simulink model "gps1"  (Simulink 7.5)
settings: Solver=ode45  StartTime=0.0  StopTime=10.0  RelTol=1e-3
undefined symbols (not defined in the file or in its folder): magnitude, serial
libraries: dspsrcs4 x32, dspxfrm3 x4, dsparch4 x2, powerlib_extras x2, dspsigops x2, instrumentlib x2, tiiqmathlib x1
settings Model: Creator=sisa  LastModifiedBy=SISA

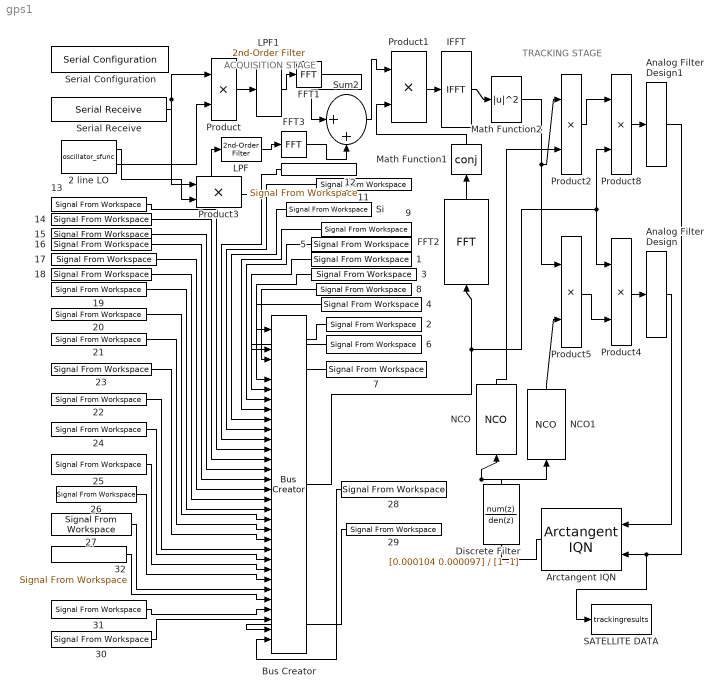
== system gps1 ==
  note: ACQUISITION STAGE
  note: TRACKING STAGE
  1 : dspsrcs4/Signal From Workspace  SystemSampleTime=-1  X=PN07  Ts=1  nsamps=1  OutputAfterFinalValue=Setting to zero  ignoreOrWarnInputAndFrameLengths=off
  11 : dspsrcs4/Signal From Workspace  SystemSampleTime=-1  X=PN11  Ts=1  nsamps=1  OutputAfterFinalValue=Setting to zero  ignoreOrWarnInputAndFrameLengths=off
  12 : dspsrcs4/Signal From Workspace  SystemSampleTime=-1  X=PN12  Ts=1  nsamps=1  OutputAfterFinalValue=Setting to zero  ignoreOrWarnInputAndFrameLengths=off
  13 : dspsrcs4/Signal From Workspace  SystemSampleTime=-1  X=PN13  Ts=1  nsamps=1  OutputAfterFinalValue=Setting to zero  ignoreOrWarnInputAndFrameLengths=off
  14 : dspsrcs4/Signal From Workspace  SystemSampleTime=-1  X=PN14  Ts=1  nsamps=1  OutputAfterFinalValue=Setting to zero  ignoreOrWarnInputAndFrameLengths=off
  15 : dspsrcs4/Signal From Workspace  SystemSampleTime=-1  X=PN15  Ts=1  nsamps=1  OutputAfterFinalValue=Setting to zero  ignoreOrWarnInputAndFrameLengths=off
  16 : dspsrcs4/Signal From Workspace  SystemSampleTime=-1  X=PN16  Ts=1  nsamps=1  OutputAfterFinalValue=Setting to zero  ignoreOrWarnInputAndFrameLengths=off
  17 : dspsrcs4/Signal From Workspace  SystemSampleTime=-1  X=PN17  Ts=1  nsamps=1  OutputAfterFinalValue=Setting to zero  ignoreOrWarnInputAndFrameLengths=off
  18 : dspsrcs4/Signal From Workspace  SystemSampleTime=-1  X=PN18  Ts=1  nsamps=1  OutputAfterFinalValue=Setting to zero  ignoreOrWarnInputAndFrameLengths=off
  19 : dspsrcs4/Signal From Workspace  SystemSampleTime=-1  X=PN19  Ts=1  nsamps=1  OutputAfterFinalValue=Setting to zero  ignoreOrWarnInputAndFrameLengths=off
  2 : dspsrcs4/Signal From Workspace  SystemSampleTime=-1  X=PN03  Ts=1  nsamps=1  OutputAfterFinalValue=Setting to zero  ignoreOrWarnInputAndFrameLengths=off
  2 line LO : M-S-Function  FunctionName=oscillator_sfunc  Parameters=1/38192000
  20 : dspsrcs4/Signal From Workspace  SystemSampleTime=-1  X=PN20  Ts=1  nsamps=1  OutputAfterFinalValue=Setting to zero  ignoreOrWarnInputAndFrameLengths=off
  21 : dspsrcs4/Signal From Workspace  SystemSampleTime=-1  X=PN21  Ts=1  nsamps=1  OutputAfterFinalValue=Setting to zero  ignoreOrWarnInputAndFrameLengths=off
  22 : dspsrcs4/Signal From Workspace  SystemSampleTime=-1  X=PN23  Ts=1  nsamps=1  OutputAfterFinalValue=Setting to zero  ignoreOrWarnInputAndFrameLengths=off
  23 : dspsrcs4/Signal From Workspace  SystemSampleTime=-1  X=PN22  Ts=1  nsamps=1  OutputAfterFinalValue=Setting to zero  ignoreOrWarnInputAndFrameLengths=off
  24 : dspsrcs4/Signal From Workspace  SystemSampleTime=-1  X=PN24  Ts=1  nsamps=1  OutputAfterFinalValue=Setting to zero  ignoreOrWarnInputAndFrameLengths=off
  25 : dspsrcs4/Signal From Workspace  SystemSampleTime=-1  X=PN25  Ts=1  nsamps=1  OutputAfterFinalValue=Setting to zero  ignoreOrWarnInputAndFrameLengths=off
  26 : dspsrcs4/Signal From Workspace  SystemSampleTime=-1  X=PN26  Ts=1  nsamps=1  OutputAfterFinalValue=Setting to zero  ignoreOrWarnInputAndFrameLengths=off
  27 : dspsrcs4/Signal From Workspace  SystemSampleTime=-1  X=PN27  Ts=1  nsamps=1  OutputAfterFinalValue=Setting to zero  ignoreOrWarnInputAndFrameLengths=off
  28 : dspsrcs4/Signal From Workspace  SystemSampleTime=-1  X=PN28  Ts=1  nsamps=1  OutputAfterFinalValue=Setting to zero  ignoreOrWarnInputAndFrameLengths=off
  29 : dspsrcs4/Signal From Workspace  SystemSampleTime=-1  X=PN29  Ts=1  nsamps=1  OutputAfterFinalValue=Setting to zero  ignoreOrWarnInputAndFrameLengths=off
  3 : dspsrcs4/Signal From Workspace  SystemSampleTime=-1  X=PN06  Ts=1  nsamps=1  OutputAfterFinalValue=Setting to zero  ignoreOrWarnInputAndFrameLengths=off
  30 : dspsrcs4/Signal From Workspace  SystemSampleTime=-1  X=PN30  Ts=1  nsamps=1  OutputAfterFinalValue=Setting to zero  ignoreOrWarnInputAndFrameLengths=off
  31 : dspsrcs4/Signal From Workspace  SystemSampleTime=-1  X=PN31  Ts=1  nsamps=1  OutputAfterFinalValue=Setting to zero  ignoreOrWarnInputAndFrameLengths=off
  32 : dspsrcs4/Signal From Workspace  SystemSampleTime=-1  X=PN32  Ts=1  nsamps=1  OutputAfterFinalValue=Setting to zero  ignoreOrWarnInputAndFrameLengths=off
  4 : dspsrcs4/Signal From Workspace  SystemSampleTime=-1  X=PN04  Ts=1  nsamps=1  OutputAfterFinalValue=Setting to zero  ignoreOrWarnInputAndFrameLengths=off
  5 : dspsrcs4/Signal From Workspace  SystemSampleTime=-1  X=PN08  Ts=1  nsamps=1  OutputAfterFinalValue=Setting to zero  ignoreOrWarnInputAndFrameLengths=off
  6 : dspsrcs4/Signal From Workspace  SystemSampleTime=-1  X=PN02  Ts=1  nsamps=1  OutputAfterFinalValue=Setting to zero  ignoreOrWarnInputAndFrameLengths=off
  7 : dspsrcs4/Signal From Workspace  SystemSampleTime=-1  X=PN01  Ts=1  nsamps=1  OutputAfterFinalValue=Setting to zero  ignoreOrWarnInputAndFrameLengths=off
  8 : dspsrcs4/Signal From Workspace  SystemSampleTime=-1  X=PN05  Ts=1  nsamps=1  OutputAfterFinalValue=Setting to zero  ignoreOrWarnInputAndFrameLengths=off
  9 : dspsrcs4/Signal From Workspace  SystemSampleTime=-1  X=PN09  Ts=1  nsamps=1  OutputAfterFinalValue=Setting to zero  ignoreOrWarnInputAndFrameLengths=off
  Analog Filter Design : dsparch4/Analog Filter Design  method=Butterworth  filttype=Lowpass  N=8  Wlo=30  Whi=80  Rp=2  Rs=40
  Analog Filter Design1 : dsparch4/Analog Filter Design  method=Chebyshev I  filttype=Lowpass  N=8  Wlo=30  Whi=80  Rp=2  Rs=40
  Arctangent IQN : tiiqmathlib/Arctangent IQN  tanOption=atan2PU (per unit)
  Bus Creator : BusCreator  Inputs=32  UseBusObject=on
  Discrete Filter : DiscreteFilter  Numerator=[0.000104 0.000097]  Denominator=[1 -1]  SampleTime=1
  FFT1 : dspxfrm3/FFT  DialogController=dspDDGCreate  DialogControllerArgs=DataTag0  CompMethod=Table lookup  TableOpt=NEW  TableOptActive=Speed  BitRevOrder=off  InheritFFTLength=on  FFTLength=64  SkipNorm=off  firstCoeffDataTypeStr=Inherit: Same word length as input  firstCoeffLastDataTypeStr=Inherit: Same word length as input  outputMin=[]  outputMax=[]  roundingMode=Floor  overflowMode=off
  FFT2 : dspxfrm3/FFT  DialogController=dspDDGCreate  DialogControllerArgs=DataTag1  CompMethod=Table lookup  TableOpt=NEW  TableOptActive=Speed  BitRevOrder=off  InheritFFTLength=on  FFTLength=64  SkipNorm=off  firstCoeffDataTypeStr=Inherit: Same word length as input  firstCoeffLastDataTypeStr=Inherit: Same word length as input  outputMin=[]  outputMax=[]  roundingMode=Floor  overflowMode=off
  FFT3 : dspxfrm3/FFT  DialogController=dspDDGCreate  DialogControllerArgs=DataTag2  CompMethod=Table lookup  TableOpt=NEW  TableOptActive=Speed  BitRevOrder=off  InheritFFTLength=on  FFTLength=64  SkipNorm=off  firstCoeffDataTypeStr=Inherit: Same word length as input  firstCoeffLastDataTypeStr=Inherit: Same word length as input  outputMin=[]  outputMax=[]  roundingMode=Floor  overflowMode=off
  IFFT : dspxfrm3/IFFT  DialogController=dspDDGCreate  DialogControllerArgs=DataTag3  CompMethod=Table lookup  TableOpt=NEW  TableOptActive=Speed  BitRevOrder=on  cs_in=off  SkipNorm=off  InheritFFTLength=on  FFTLength=1024  mode=Complex  outSamplingMode=Sample based  firstCoeffDataTypeStr=Inherit: Same word length as input  firstCoeffLastDataTypeStr=Inherit: Same word length as input  outputMin=[]  outputMax=[]  roundingMode=Floor  overflowMode=off
  LPF : powerlib_extras/Control  Blocks/2nd-Order Filter  DialogController=POWERSYS.PowerSysDialog  SystemSampleTime=-1  FilterType=Lowpass  Fo=15  Zeta=0.707  Initialize=off  Vac_Init=[1 45 60]  Vdc_Init=-0.5  PlotResponse=off  param1=[1 500 1]
  LPF1 : powerlib_extras/Control  Blocks/2nd-Order Filter  DialogController=POWERSYS.PowerSysDialog  SystemSampleTime=-1  FilterType=Lowpass  Fo=15  Zeta=0.707  Initialize=off  Vac_Init=[1 45 60]  Vdc_Init=-0.5  PlotResponse=off  param1=[1 500 1]
  Math Function1 : Math  Operator=conj  OutputSignalType=complex  OutDataType=fixdt(1, 16)  OutScaling=2^0  SaturateOnIntegerOverflow=on
  Math Function2 : Math  Operator=magnitude^2  OutputSignalType=real  OutDataType=fixdt(1, 16)  OutScaling=2^0  SaturateOnIntegerOverflow=on
  NCO : dspsigops/NCO  DialogController=dspdialog.NCO  AccIncSrc=Input port  AccInc=100  PhaseOffsetSrc=Specify via dialog  PhaseOffset=0  AccumWL=16  HasDither=on  DitherWL=4  PNgeneratorLength=19  HasPhaseQuantizer=on  TableDepth=12  HasOutputPhaseError=off  Formula=Cosine  DataType=Binary point scaling  OutputWL=16  OutputFL=14  CompMethod=Table lookup (no interpolation)  SampleTime=1  SamplesPerFrame=1
  NCO1 : dspsigops/NCO  DialogController=dspdialog.NCO  AccIncSrc=Input port  AccInc=100  PhaseOffsetSrc=Specify via dialog  PhaseOffset=0  AccumWL=16  HasDither=on  DitherWL=4  PNgeneratorLength=19  HasPhaseQuantizer=on  TableDepth=12  HasOutputPhaseError=off  Formula=Sine  DataType=Binary point scaling  OutputWL=16  OutputFL=14  CompMethod=Table lookup (no interpolation)  SampleTime=1  SamplesPerFrame=1
  Product{,1..5,8} (7 alike) : Product  OutDataType=fixdt(1, 16)  OutScaling=2^0  RndMeth=Zero
  SATELLITE DATA : ToWorkspace  VariableName=trackingresults  SampleTime=-1  SaveFormat=Array
      settings: MaxDataPoints=1023
  Serial Configuration : instrumentlib/Serial Configuration  Priority=-200000  DialogController=instrumentcreatedialog  DialogControllerArgs=DataTag4  ComPortMenu=COM1  ComPort=COM1  ObjConstructor=serial('COM1');  BaudRate=9600  DataBits=8  Parity=none  StopBits=1  FlowControl=none  Timeout=10  ByteOrder=LittleEndian
  Serial Receive : instrumentlib/Serial Receive  DialogController=instrumentcreatedialog  DialogControllerArgs=DataTag5  ComPortMenu=COM1  ComPort=COM1  ObjConstructor=serial('COM1');  Header=none  Terminator=<none>  DataSize="[1  1]"  DataType=uint8  EnableBlockingMode=on  ActionDataUnavailable=Output last received value  CustomValue=0  SampleTime=0.01
  Si : dspsrcs4/Signal From Workspace  SystemSampleTime=-1  X=PN10  Ts=1  nsamps=1  OutputAfterFinalValue=Setting to zero  ignoreOrWarnInputAndFrameLengths=off
  Sum2 : Sum  Inputs=|++  OutDataType=fixdt(1, 16)  OutScaling=2^0
  wires:
  Serial Receive/1 -> Product/1, Product3/1
  FFT2/1 -> Math Function1/1
  2 line LO/1 -> Product3/2
  2 line LO/2 -> Product/2
  9/1 -> Bus Creator/9
  Si/1 -> Bus Creator/10
  11/1 -> Bus Creator/11
  12/1 -> Bus Creator/12
  13/1 -> Bus Creator/13
  14/1 -> Bus Creator/14
  15/1 -> Bus Creator/15
  16/1 -> Bus Creator/16
  17/1 -> Bus Creator/17
  18/1 -> Bus Creator/18
  19/1 -> Bus Creator/19
  28/1 -> Bus Creator/32
  32/1 -> Bus Creator/28
  20/1 -> Bus Creator/20
  21/1 -> Bus Creator/21
  23/1 -> Bus Creator/22
  22/1 -> Bus Creator/23
  24/1 -> Bus Creator/24
  25/1 -> Bus Creator/25
  26/1 -> Bus Creator/26
  27/1 -> Bus Creator/27
  NCO/1 -> Product2/2
  Product4/1 -> Analog Filter Design/1
  Product8/1 -> Analog Filter Design1/1
  Product2/1 -> Product8/1
  NCO1/1 -> Product5/2
  29/1 -> Bus Creator/31
  30/1 -> Bus Creator/30
  31/1 -> Bus Creator/29
  Math Function2/1 -> Product5/1, Product2/1
  Arctangent IQN/1 -> Discrete Filter/1
  Discrete Filter/1 -> NCO/1, NCO1/1
  Math Function1/1 -> Product1/2
  5/1 -> Bus Creator/8
  1/1 -> Bus Creator/7
  3/1 -> Bus Creator/6
  8/1 -> Bus Creator/4
  7/1 -> Bus Creator/5
  6/1 -> Bus Creator/3
  2/1 -> Bus Creator/2
  4/1 -> Bus Creator/1
  Bus Creator/1 -> FFT2/1, Product8/2, Product4/1
  Product5/1 -> Product4/2
  Analog Filter Design/1 -> Arctangent IQN/1
  Analog Filter Design1/1 -> Arctangent IQN/2, SATELLITE DATA/1
  Product3/1 -> LPF/1
  Product/1 -> LPF1/1
  Sum2/1 -> Product1/1
  LPF1/1 -> FFT1/1
  FFT1/1 -> Sum2/1
  FFT3/1 -> Sum2/2
  LPF/1 -> FFT3/1
  IFFT/1 -> Math Function2/1
  Product1/1 -> IFFT/1
